simulink model "nine"  (R2020b)
settings: Solver=VariableStepAuto  StartTime=0.0  StopTime=10.0  RelTol=1e-3
undefined symbols (not defined in the file): K
settings Model: Creator=priyaD  LastModifiedBy=priyaD

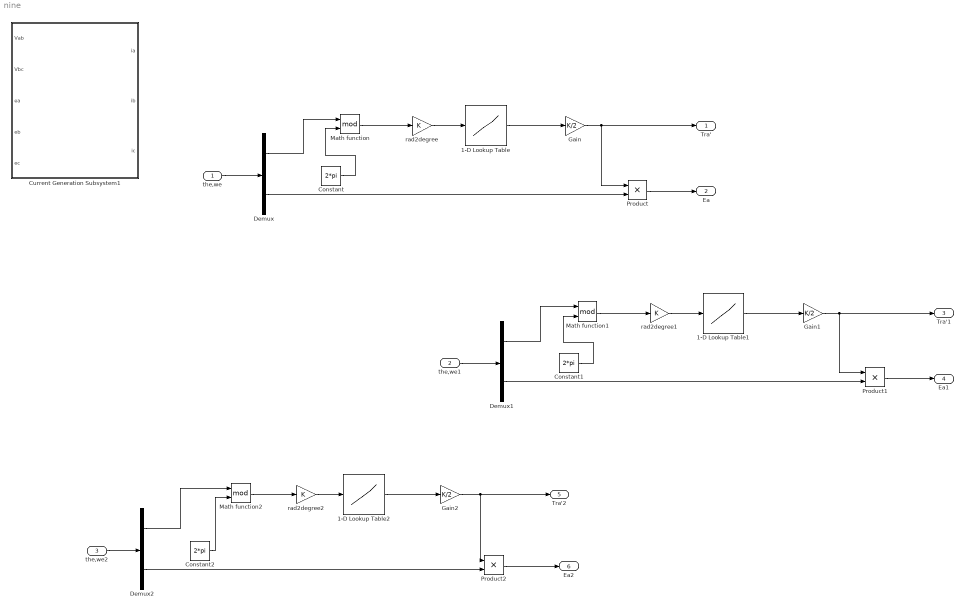
== system nine ==
  the,we : Inport
  the,we1 : Inport  Port=2
  the,we2 : Inport  Port=3
  1-D Lookup Table : Lookup_n-D  NumberOfTableDimensions=1  BreakpointsForDimension1=[-5:5]  Table=tanh([-5:5])  InternalRulePriority=Speed  RndMeth=Simplest  InputSameDT=on
  1-D Lookup Table1 : Lookup_n-D  NumberOfTableDimensions=1  BreakpointsForDimension1=[-5:5]  Table=tanh([-5:5])  InternalRulePriority=Speed  RndMeth=Simplest  InputSameDT=on
  1-D Lookup Table2 : Lookup_n-D  NumberOfTableDimensions=1  BreakpointsForDimension1=[-5:5]  Table=tanh([-5:5])  InternalRulePriority=Speed  RndMeth=Simplest  InputSameDT=on
  Constant : Constant  Value=2*pi
  Constant1 : Constant  Value=2*pi
  Constant2 : Constant  Value=2*pi
  Current Generation Subsystem1 : Subsystem
  Demux : Demux  Outputs=2
  Demux1 : Demux  Outputs=2
  Demux2 : Demux  Outputs=2
  Gain : Gain  Gain=K/2
  Gain1 : Gain  Gain=K/2
  Gain2 : Gain  Gain=K/2
  Math function : Math  Operator=mod  SaturateOnIntegerOverflow=on
  Math function1 : Math  Operator=mod  SaturateOnIntegerOverflow=on
  Math function2 : Math  Operator=mod  SaturateOnIntegerOverflow=on
  Product : Product
  Product1 : Product
  Product2 : Product
  rad2degree : Gain  Gain=K
  rad2degree1 : Gain  Gain=K
  rad2degree2 : Gain  Gain=K
  Tra' : Outport
  Ea : Outport  Port=2
  Tra'1 : Outport  Port=3
  Ea1 : Outport  Port=4
  Tra'2 : Outport  Port=5
  Ea2 : Outport  Port=6
  wires:
  the,we/1 -> Demux/1
  Demux/1 -> Math function/1
  Constant/1 -> Math function/2
  Math function/1 -> rad2degree/1
  rad2degree/1 -> 1-D Lookup Table/1
  1-D Lookup Table/1 -> Gain/1
  Demux/2 -> Product/2
  Gain/1 -> Product/1, Tra'/1
  Product/1 -> Ea/1
  the,we1/1 -> Demux1/1
  1-D Lookup Table1/1 -> Gain1/1
  Constant1/1 -> Math function1/2
  Demux1/2 -> Product1/2
  Gain1/1 -> Product1/1, Tra'1/1
  Math function1/1 -> rad2degree1/1
  Demux1/1 -> Math function1/1
  rad2degree1/1 -> 1-D Lookup Table1/1
  Product1/1 -> Ea1/1
  the,we2/1 -> Demux2/1
  1-D Lookup Table2/1 -> Gain2/1
  Constant2/1 -> Math function2/2
  Demux2/2 -> Product2/2
  Gain2/1 -> Tra'2/1, Product2/1
  Math function2/1 -> rad2degree2/1
  Demux2/1 -> Math function2/1
  rad2degree2/1 -> 1-D Lookup Table2/1
  Product2/1 -> Ea2/1

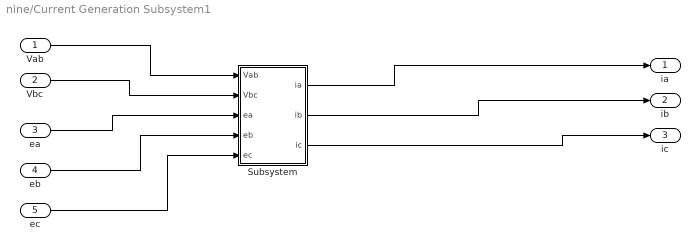
== system nine/Current Generation Subsystem1 ==
  Vab : Inport
  Vbc : Inport  Port=2
  ea : Inport  Port=3
  eb : Inport  Port=4
  ec : Inport  Port=5
  Subsystem : Subsystem
  ia : Outport
  ib : Outport  Port=2
  ic : Outport  Port=3
  wires:
  Vbc/1 -> Subsystem/2(Vbc)
  Vab/1 -> Subsystem/1(Vab)
  Subsystem/1(ia) -> ia/1
  ea/1 -> Subsystem/3(ea)
  ec/1 -> Subsystem/5(ec)
  Subsystem/3(ic) -> ic/1
  Subsystem/2(ib) -> ib/1
  eb/1 -> Subsystem/4(eb)

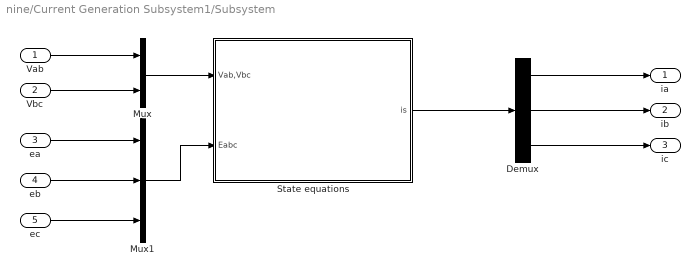
== system nine/Current Generation Subsystem1/Subsystem ==
  Vab : Inport
  Vbc : Inport  Port=2
  ea : Inport  Port=3
  eb : Inport  Port=4
  ec : Inport  Port=5
  Demux : Demux  Outputs=3
  Mux : Mux  Inputs=2
  Mux1 : Mux  Inputs=3
  State equations : Subsystem
  ia : Outport
  ib : Outport  Port=2
  ic : Outport  Port=3
  wires:
  Demux/3 -> ic/1
  Mux/1 -> State equations/1(Vab,Vbc)
  State equations/1(is) -> Demux/1
  ea/1 -> Mux1/1
  Demux/1 -> ia/1
  ec/1 -> Mux1/3
  eb/1 -> Mux1/2
  Mux1/1 -> State equations/2(Eabc)
  Demux/2 -> ib/1
  Vbc/1 -> Mux/2
  Vab/1 -> Mux/1

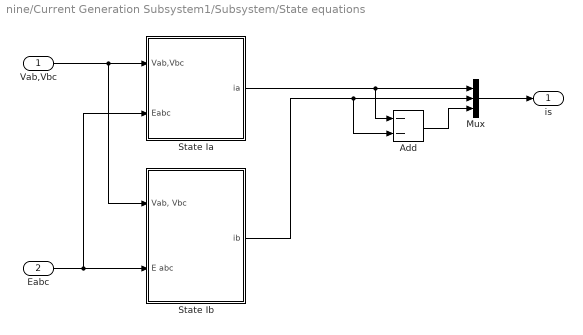
== system nine/Current Generation Subsystem1/Subsystem/State equations ==
  Vab,Vbc : Inport
  Eabc : Inport  Port=2
  Add : Sum  Inputs=--
  Mux : Mux  Inputs=3
  State Ia : Subsystem
  State Ib : Subsystem
  is : Outport
  wires:
  Vab,Vbc/1 -> State Ib/1("Vab, Vbc"), State Ia/1(Vab,Vbc)
  State Ia/1(ia) -> Add/1, Mux/1
  Add/1 -> Mux/3
  State Ib/1(ib) -> Add/2, Mux/2
  Eabc/1 -> State Ib/2(E abc), State Ia/2(Eabc)
  Mux/1 -> is/1

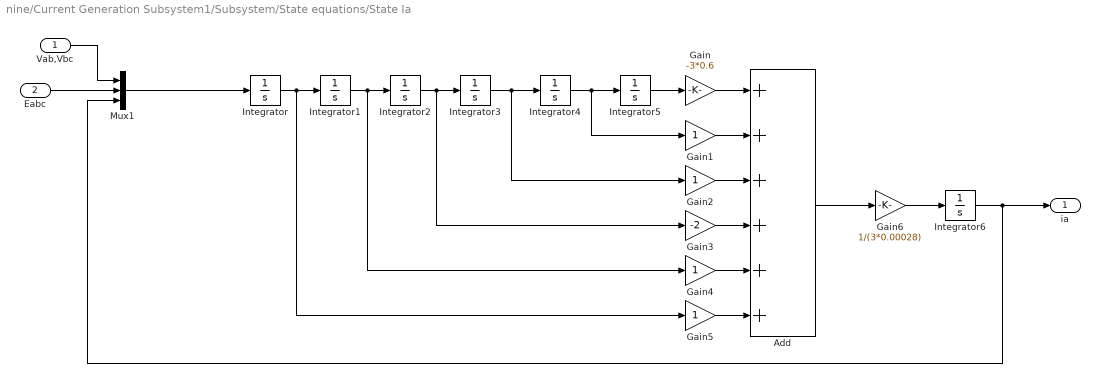
== system nine/Current Generation Subsystem1/Subsystem/State equations/State Ia ==
  Vab,Vbc : Inport
  Eabc : Inport  Port=2
  Add : Sum  Inputs=++++++
  Gain : Gain  Gain=-3*0.6
  Gain{1..2,4..5} (4 alike) : Gain
  Gain3 : Gain  Gain=-2
  Gain6 : Gain  Gain=1/(3*0.00028)
  Integrator{,1..6} (7 alike) : Integrator
  Mux1 : Mux  Inputs=3
  ia : Outport
  wires:
  Gain1/1 -> Add/2
  Gain3/1 -> Add/4
  Integrator3/1 -> Gain2/1, Integrator4/1
  Mux1/1 -> Integrator/1
  Vab,Vbc/1 -> Mux1/1
  Integrator1/1 -> Gain4/1, Integrator2/1
  Gain5/1 -> Add/6
  Integrator6/1 -> ia/1, Mux1/3
  Integrator2/1 -> Gain3/1, Integrator3/1
  Integrator4/1 -> Gain1/1, Integrator5/1
  Add/1 -> Gain6/1
  Gain6/1 -> Integrator6/1
  Gain/1 -> Add/1
  Integrator/1 -> Gain5/1, Integrator1/1
  Eabc/1 -> Mux1/2
  Integrator5/1 -> Gain/1
  Gain4/1 -> Add/5
  Gain2/1 -> Add/3

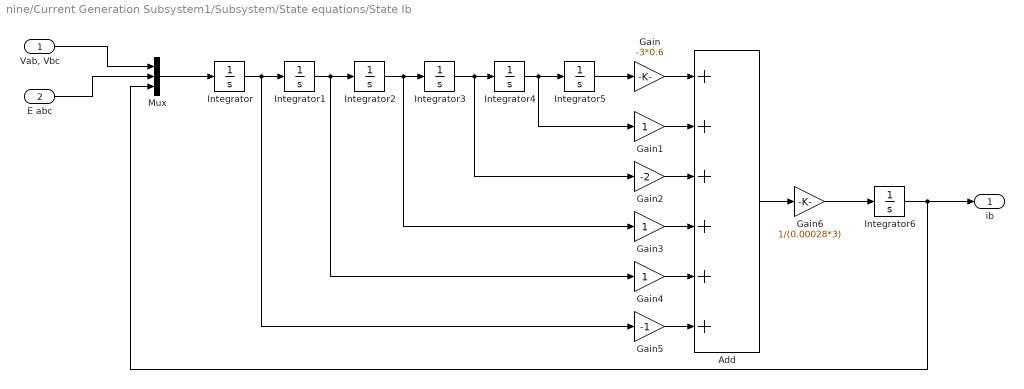
== system nine/Current Generation Subsystem1/Subsystem/State equations/State Ib ==
  "Vab, Vbc" : Inport
  E abc : Inport  Port=2
  Add : Sum  Inputs=++++++
  Gain : Gain  Gain=-3*0.6
  Gain1 : Gain
  Gain2 : Gain  Gain=-2
  Gain3 : Gain
  Gain4 : Gain
  Gain5 : Gain  Gain=-1
  Gain6 : Gain  Gain=1/(0.00028*3)
  Integrator{,1..6} (7 alike) : Integrator
  Mux : Mux  Inputs=3
  ib : Outport
  wires:
  E abc/1 -> Mux/2
  Gain/1 -> Add/1
  Integrator/1 -> Gain5/1, Integrator1/1
  Integrator1/1 -> Gain4/1, Integrator2/1
  Integrator2/1 -> Gain3/1, Integrator3/1
  Integrator3/1 -> Gain2/1, Integrator4/1
  Add/1 -> Gain6/1
  Gain5/1 -> Add/6
  Gain6/1 -> Integrator6/1
  Integrator6/1 -> ib/1, Mux/3
  Integrator4/1 -> Gain1/1, Integrator5/1
  Mux/1 -> Integrator/1
  Gain4/1 -> Add/5
  Gain2/1 -> Add/3
  Gain3/1 -> Add/4
  Integrator5/1 -> Gain/1
  Gain1/1 -> Add/2
  "Vab, Vbc"/1 -> Mux/1
